simulink model "ThrdRwRtStCshnFldTrgtPosSelc"  (R2018b)
settings: Solver=FixedStepDiscrete  StartTime=0.0  StopTime=10.0  FixedStep=0.01  RelTol=1e-3
undefined symbols (not defined in the file or in its folder): KeSMSw6sAcsEntryThdRwRtStCshnFldUpwdDnwdPos_Val, KeSMSw6sAcsEntryThdRwRtStCshnFldUpwdDnwdPosMax_Val, KeSMSw6sAcsEntryThdRwRtStCshnFldUpwdDnwdPosMin_Val, KeSMSw6sLugThdRwRtStCshnFldUpwdDnwdPos_Val, KeSMSw6sLugThdRwRtStCshnFldUpwdDnwdPosMax_Val, KeSMSw6sLugThdRwRtStCshnFldUpwdDnwdPosMin_Val, KeSMSwAcsEntryThdRwRtStCshnFldUpwdDnwdPos_Val, KeSMSwAcsEntryThdRwRtStCshnFldUpwdDnwdPosMax_Val, KeSMSwAcsEntryThdRwRtStCshnFldUpwdDnwdPosMin_Val, KeSMSwLugThdRwRtStCshnFldUpwdDnwdPos_Val, KeSMSwLugThdRwRtStCshnFldUpwdDnwdPosMax_Val, KeSMSwLugThdRwRtStCshnFldUpwdDnwdPosMin_Val
libraries: TrgtPosSelcLib x3
settings Model: Creator=sn2xws  LastModifiedBy=sn2xws
settings DataIOCC: SaveFormat=StructureWithTime
settings OptimizationCC: DefaultParameterBehavior=Inlined  EnhancedBackFolding=on  PassReuseOutputArgsAs=Individual arguments  ZeroExternalMemoryAtStartup=off  ZeroInternalMemoryAtStartup=off  OptimizeBlockOrder=speed  DifferentSizesBufferReuse=on  OptimizationCustomize=off
settings DebuggingCC: ParameterTunabilityLossMsg=error
settings ModelReferenceCC: ModelReferenceNumInstancesAllowed=Single
settings SFSimCC: MATLABDynamicMemAlloc=off
settings RTWCC: SystemTargetFile=autosar.tlc  GenCodeOnly=on  TemplateMakefile=ert_default_tmf  Description=AUTOSAR  GenerateReport=on  IncludeHyperlinkInReport=on  LaunchReport=on  GenerateTraceInfo=on  GenerateTraceReport=on  GenerateTraceReportSl=on  GenerateTraceReportSf=on  GenerateTraceReportEml=on
settings CodeAppCC: ForceParamTrailComments=on  IgnoreCustomStorageClasses=off  OperatorAnnotations=on  SimulinkDataObjDesc=on  SFDataObjDesc=on  InsertBlockDesc=on
settings STFCustomTargetCC: TargetLangStandard=C99 (ISO)  MultiwordLength=256  ParMdlRefBuildCompliant=on  CompOptLevelCompliant=on  IncludeMdlTerminateFcn=off  CombineOutputUpdateFcns=on  SuppressErrorStatus=on  ERTCustomFileBanners=on  SupportNonFinite=off  SupportComplex=off  SupportContinuousTime=off  SupportNonInlinedSFcns=off  RemoveResetFunc=on  MATLABClassNameForMDSCustomization=Simulink.SoftwareTarget.ERTCustomization  AutosarCompliant=on  UseToolchainInfoCompliant=on  LookupTableObjectStructAxisOrder=2,1,3,4,...  LUTObjectStructOrderEvenSpacing=Size,Table,Breakpoints  SystemTargetFile=autosar.tlc
settings ERTTargetCC: TargetLangStandard=C99 (ISO)  ConcurrentExecutionCompliant=off  IncludeMdlTerminateFcn=off  SuppressErrorStatus=on  SupportNonFinite=off  SupportComplex=off  ModelStepFunctionPrototypeControlCompliant=off  CPPClassGenCompliant=off  AutosarCompliant=on  LookupTableObjectStructAxisOrder=2,1,3,4,...  LUTObjectStructOrderEvenSpacing=Size,Table,Breakpoints  InlinedParameterPlacement=NonHierarchical  ERTCustomFileTemplate=example_file_process.tlc

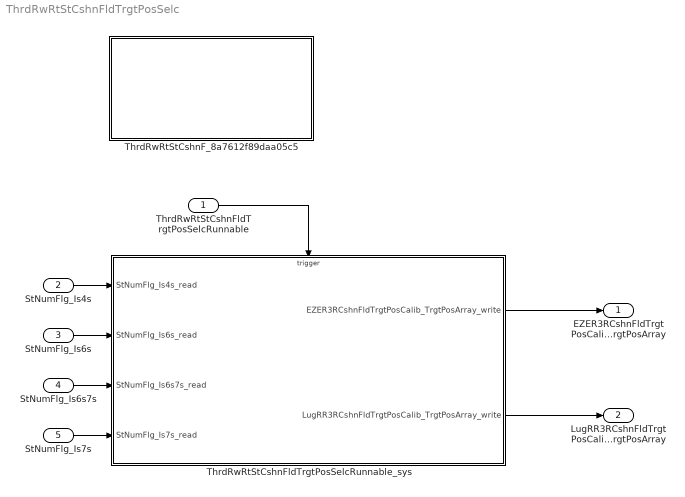
== system ThrdRwRtStCshnFldTrgtPosSelc ==
  ThrdRwRtStCshnFldTrgtPosSelcRunnable : Inport  SampleTime=0.01  OutputFunctionCall=on
  StNumFlg_Is4s : Inport  Port=2  OutDataTypeStr=boolean  PortDimensions=1
  StNumFlg_Is6s : Inport  Port=3  OutDataTypeStr=boolean  PortDimensions=1
  StNumFlg_Is6s7s : Inport  Port=4  OutDataTypeStr=boolean  PortDimensions=1
  StNumFlg_Is7s : Inport  Port=5  OutDataTypeStr=boolean  PortDimensions=1
  ThrdRwRtStCshnF_8a7612f89daa05c5 : Subsystem
  ThrdRwRtStCshnFldTrgtPosSelcRunnable_sys : Subsystem
  EZER3RCshnFldTrgtPosCalib_TrgtPosArray : Outport  Description=|  OutDataTypeStr=uint16  PortDimensions=3
      | 0:Pos
      | 1:Max
      | 2:Min
  LugRR3RCshnFldTrgtPosCalib_TrgtPosArray : Outport  Description=|  Port=2  OutDataTypeStr=uint16  PortDimensions=3
      | 0:Pos
      | 1:Max
      | 2:Min
  wires:
  StNumFlg_Is4s/1 -> ThrdRwRtStCshnFldTrgtPosSelcRunnable_sys/1(StNumFlg_Is4s_read)
  StNumFlg_Is6s/1 -> ThrdRwRtStCshnFldTrgtPosSelcRunnable_sys/2(StNumFlg_Is6s_read)
  StNumFlg_Is6s7s/1 -> ThrdRwRtStCshnFldTrgtPosSelcRunnable_sys/3(StNumFlg_Is6s7s_read)
  StNumFlg_Is7s/1 -> ThrdRwRtStCshnFldTrgtPosSelcRunnable_sys/4(StNumFlg_Is7s_read)
  ThrdRwRtStCshnFldTrgtPosSelcRunnable_sys/1(EZER3RCshnFldTrgtPosCalib_TrgtPosArray_write) -> EZER3RCshnFldTrgtPosCalib_TrgtPosArray/1
  ThrdRwRtStCshnFldTrgtPosSelcRunnable_sys/2(LugRR3RCshnFldTrgtPosCalib_TrgtPosArray_write) -> LugRR3RCshnFldTrgtPosCalib_TrgtPosArray/1
  ThrdRwRtStCshnFldTrgtPosSelcRunnable/1 -> ThrdRwRtStCshnFldTrgtPosSelcRunnable_sys/Trigger

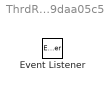
== system ThrdRwRtStCshnFldTrgtPosSelc/ThrdRwRtStCshnF_8a7612f89daa05c5 ==
  Event Listener : EventListener  EventName=reset

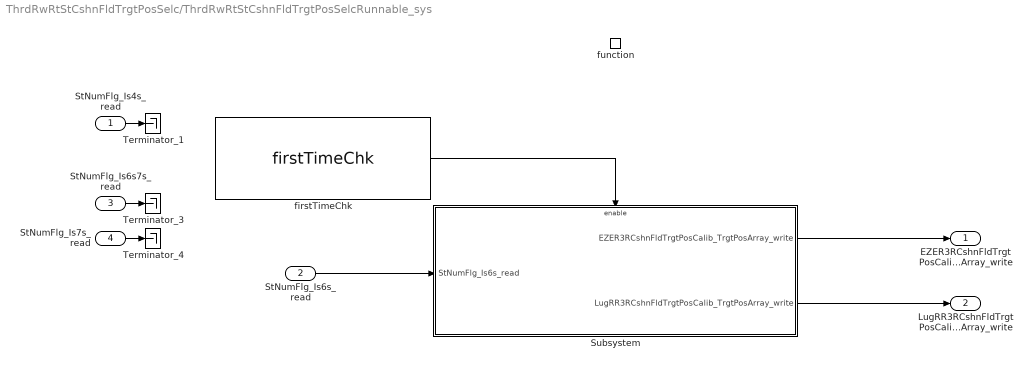
== system ThrdRwRtStCshnFldTrgtPosSelc/ThrdRwRtStCshnFldTrgtPosSelcRunnable_sys ==
  StNumFlg_Is4s_read : Inport
  StNumFlg_Is6s_read : Inport  Port=2
  StNumFlg_Is6s7s_read : Inport  Port=3
  StNumFlg_Is7s_read : Inport  Port=4
  function : TriggerPort  TriggerType=function-call  VariantControl=(inherit)  SampleTimeType=periodic  SampleTime=-1
  Subsystem : Subsystem
  Terminator_1 : Terminator
  Terminator_3 : Terminator
  Terminator_4 : Terminator
  firstTimeChk : TrgtPosSelcLib/firstTimeChk  SystemSampleTime=-1
  EZER3RCshnFldTrgtPosCalib_TrgtPosArray_write : Outport
      settings: EnsureOutportIsVirtual=on
  LugRR3RCshnFldTrgtPosCalib_TrgtPosArray_write : Outport  Port=2
      settings: EnsureOutportIsVirtual=on
  wires:
  StNumFlg_Is4s_read/1 -> Terminator_1/1
  StNumFlg_Is6s7s_read/1 -> Terminator_3/1
  StNumFlg_Is7s_read/1 -> Terminator_4/1
  StNumFlg_Is6s_read/1 -> Subsystem/1(StNumFlg_Is6s_read)
  Subsystem/1(EZER3RCshnFldTrgtPosCalib_TrgtPosArray_write) -> EZER3RCshnFldTrgtPosCalib_TrgtPosArray_write/1
  Subsystem/2(LugRR3RCshnFldTrgtPosCalib_TrgtPosArray_write) -> LugRR3RCshnFldTrgtPosCalib_TrgtPosArray_write/1
  firstTimeChk/1 -> Subsystem/Enable

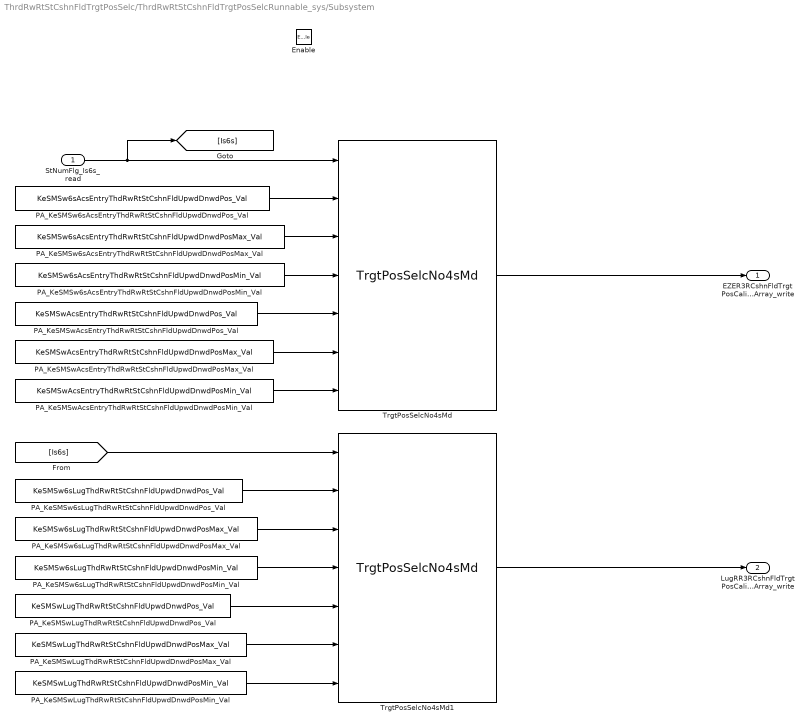
== system ThrdRwRtStCshnFldTrgtPosSelc/ThrdRwRtStCshnFldTrgtPosSelcRunnable_sys/Subsystem ==
  StNumFlg_Is6s_read : Inport
  Enable : EnablePort
  PA_KeSMSw6sAcsEntryThdRwRtStCshnFldUpwdDnwdPosMax_Val : Constant  Value=KeSMSw6sAcsEntryThdRwRtStCshnFldUpwdDnwdPosMax_Val
  PA_KeSMSw6sAcsEntryThdRwRtStCshnFldUpwdDnwdPosMin_Val : Constant  Value=KeSMSw6sAcsEntryThdRwRtStCshnFldUpwdDnwdPosMin_Val
  PA_KeSMSw6sAcsEntryThdRwRtStCshnFldUpwdDnwdPos_Val : Constant  Value=KeSMSw6sAcsEntryThdRwRtStCshnFldUpwdDnwdPos_Val
  PA_KeSMSw6sLugThdRwRtStCshnFldUpwdDnwdPosMax_Val : Constant  Value=KeSMSw6sLugThdRwRtStCshnFldUpwdDnwdPosMax_Val
  PA_KeSMSw6sLugThdRwRtStCshnFldUpwdDnwdPosMin_Val : Constant  Value=KeSMSw6sLugThdRwRtStCshnFldUpwdDnwdPosMin_Val
  PA_KeSMSw6sLugThdRwRtStCshnFldUpwdDnwdPos_Val : Constant  Value=KeSMSw6sLugThdRwRtStCshnFldUpwdDnwdPos_Val
  PA_KeSMSwAcsEntryThdRwRtStCshnFldUpwdDnwdPosMax_Val : Constant  Value=KeSMSwAcsEntryThdRwRtStCshnFldUpwdDnwdPosMax_Val
  PA_KeSMSwAcsEntryThdRwRtStCshnFldUpwdDnwdPosMin_Val : Constant  Value=KeSMSwAcsEntryThdRwRtStCshnFldUpwdDnwdPosMin_Val
  PA_KeSMSwAcsEntryThdRwRtStCshnFldUpwdDnwdPos_Val : Constant  Value=KeSMSwAcsEntryThdRwRtStCshnFldUpwdDnwdPos_Val
  PA_KeSMSwLugThdRwRtStCshnFldUpwdDnwdPosMax_Val : Constant  Value=KeSMSwLugThdRwRtStCshnFldUpwdDnwdPosMax_Val
  PA_KeSMSwLugThdRwRtStCshnFldUpwdDnwdPosMin_Val : Constant  Value=KeSMSwLugThdRwRtStCshnFldUpwdDnwdPosMin_Val
  PA_KeSMSwLugThdRwRtStCshnFldUpwdDnwdPos_Val : Constant  Value=KeSMSwLugThdRwRtStCshnFldUpwdDnwdPos_Val
  TrgtPosSelcNo4sMd : TrgtPosSelcLib/TrgtPosSelcNo4sMd  SystemSampleTime=-1
  TrgtPosSelcNo4sMd1 : TrgtPosSelcLib/TrgtPosSelcNo4sMd  SystemSampleTime=-1
  EZER3RCshnFldTrgtPosCalib_TrgtPosArray_write : Outport
      settings: EnsureOutportIsVirtual=on
  LugRR3RCshnFldTrgtPosCalib_TrgtPosArray_write : Outport  Port=2
      settings: EnsureOutportIsVirtual=on
  wires:
  StNumFlg_Is6s_read/1 -> [Is6s], TrgtPosSelcNo4sMd/1
  TrgtPosSelcNo4sMd/1 -> EZER3RCshnFldTrgtPosCalib_TrgtPosArray_write/1
  TrgtPosSelcNo4sMd1/1 -> LugRR3RCshnFldTrgtPosCalib_TrgtPosArray_write/1
  PA_KeSMSw6sAcsEntryThdRwRtStCshnFldUpwdDnwdPosMax_Val/1 -> TrgtPosSelcNo4sMd/3
  PA_KeSMSw6sAcsEntryThdRwRtStCshnFldUpwdDnwdPos_Val/1 -> TrgtPosSelcNo4sMd/2
  PA_KeSMSw6sAcsEntryThdRwRtStCshnFldUpwdDnwdPosMin_Val/1 -> TrgtPosSelcNo4sMd/4
  PA_KeSMSwAcsEntryThdRwRtStCshnFldUpwdDnwdPosMax_Val/1 -> TrgtPosSelcNo4sMd/6
  PA_KeSMSwAcsEntryThdRwRtStCshnFldUpwdDnwdPosMin_Val/1 -> TrgtPosSelcNo4sMd/7
  PA_KeSMSwAcsEntryThdRwRtStCshnFldUpwdDnwdPos_Val/1 -> TrgtPosSelcNo4sMd/5
  [Is6s] -> TrgtPosSelcNo4sMd1/1
  PA_KeSMSw6sLugThdRwRtStCshnFldUpwdDnwdPosMax_Val/1 -> TrgtPosSelcNo4sMd1/3
  PA_KeSMSw6sLugThdRwRtStCshnFldUpwdDnwdPos_Val/1 -> TrgtPosSelcNo4sMd1/2
  PA_KeSMSw6sLugThdRwRtStCshnFldUpwdDnwdPosMin_Val/1 -> TrgtPosSelcNo4sMd1/4
  PA_KeSMSwLugThdRwRtStCshnFldUpwdDnwdPosMin_Val/1 -> TrgtPosSelcNo4sMd1/7
  PA_KeSMSwLugThdRwRtStCshnFldUpwdDnwdPosMax_Val/1 -> TrgtPosSelcNo4sMd1/6
  PA_KeSMSwLugThdRwRtStCshnFldUpwdDnwdPos_Val/1 -> TrgtPosSelcNo4sMd1/5
